simulink model "LinearizedModel60"  (R2020b)
settings: Solver=VariableStepAuto  StartTime=0.0  StopTime=150  RelTol=1e-3
values from neighbouring files (symbols this model uses):
  A = sys.a    [LinMod60rpmForLqr.m]    (also in SymbolicEvaluationXhat.m = double(A))
  B = sys.b    [LinMod60rpmForLqr.m]    (also in OtterFunction_EKF.m = 1.08; OtterFunction_lqr.m = 1.08)
  C = sys.c    [LinMod60rpmForLqr.m]    (also in OtterFunction_EKF.m = CRB + CA; OtterFunction_lqr.m = CRB + CA)
  D = sys.d    [LinMod60rpmForLqr.m]
  u0 = [60 60]'    [LinMod60rpmForLqr.m]
  x0 = OpTrim60.states.x    [LinMod60rpmForLqr.m]
libraries: simulink x1, mssSimulink x1
settings Model: Creator=rapha  LastModifiedBy=rapha

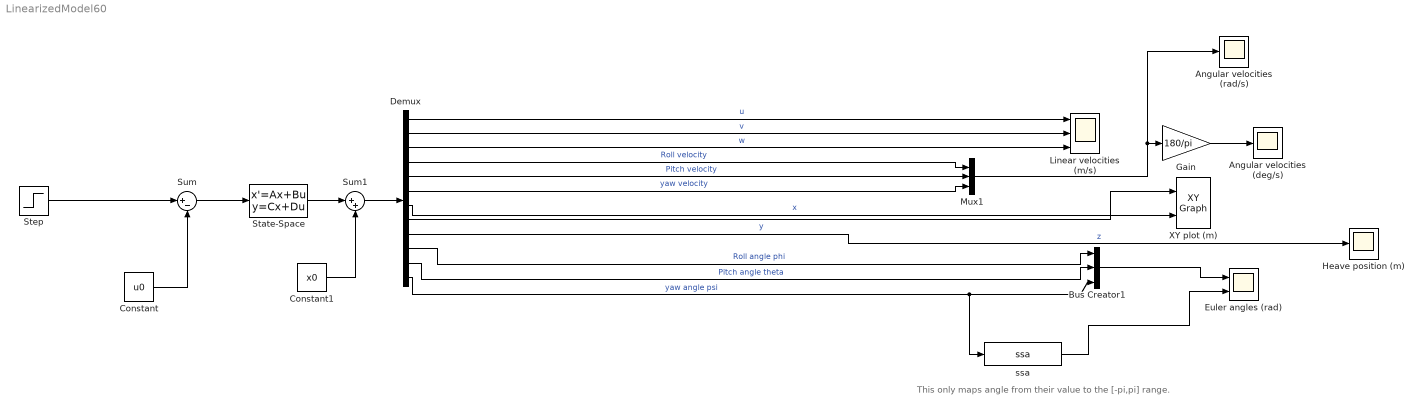
== system LinearizedModel60 ==
  note: This only maps angle from their value to the [-pi,pi] range.
  Angular velocities (deg/s) : Scope
  Angular velocities (rad/s) : Scope
  Bus Creator1 : BusCreator  Inputs=3
  Constant : Constant  Value=u0
  Constant1 : Constant  Value=x0
  Demux : Demux  Outputs=12
  Euler angles (rad) : Scope  NumInputPorts=2
  Gain : Gain  Gain=180/pi
  Heave position (m) : Scope
  Linear velocities (m/s) : Scope  NumInputPorts=3
  Mux1 : Mux  Inputs=3
  State-Space : StateSpace  A=A  B=B  C=C  D=D  InitialCondition=0
  Step : Step  Before=[60 60]  After=[70 60]  SampleTime=0
  Sum : Sum  Inputs=|+-
  Sum1 : Sum  Inputs=|++
  XY plot (m) : simulink/Sinks/XY Graph  xmin=-70  xmax=70  ymin=-70  ymax=70  st=0.01
  "ssa   " : mssSimulink/Utilities/Math Operations/ssa  SystemSampleTime=-1  VariantActivationTime=update diagram  Latency=0  AutoFrameSizeCalculation=off
  wires:
  Sum/1 -> State-Space/1
  Constant/1 -> Sum/2
  Step/1 -> Sum/1
  State-Space/1 -> Sum1/1
  Constant1/1 -> Sum1/2
  Sum1/1 -> Demux/1
  "ssa   "/1 -> Euler angles (rad)/2
  Demux/3 -> Linear velocities (m/s)/3  "w"
  Demux/2 -> Linear velocities (m/s)/2  "v"
  Demux/11 -> Bus Creator1/2  "Pitch angle theta"
  Demux/8 -> XY plot (m)/1  "y"
  Demux/5 -> Mux1/2  "Pitch velocity"
  Demux/9 -> Heave position (m)/1  "z"
  Demux/7 -> XY plot (m)/2  "x"
  Demux/4 -> Mux1/1  "Roll velocity"
  Mux1/1 -> Angular velocities (rad/s)/1, Gain/1
  Gain/1 -> Angular velocities (deg/s)/1
  Demux/10 -> Bus Creator1/1  "Roll angle phi"
  Bus Creator1/1 -> Euler angles (rad)/1
  Demux/12 -> Bus Creator1/3, "ssa   "/1  "yaw angle psi"
  Demux/1 -> Linear velocities (m/s)/1  "u"
  Demux/6 -> Mux1/3  "yaw velocity"
